simulink model "SerialWriteText"  (R2018a)
settings: Solver=FixedStepAuto  StartTime=0.0  StopTime=5  FixedStep=.1  RelTol=1e-3
libraries: arduinolib x1
settings Model: ExtModeTrigDuration=2  Creator=jonathancoulter  LastModifiedBy=jonathancoulter
settings OptimizationCC: UseFloatMulNetSlope=on  PassReuseOutputArgsThreshold=0  EfficientFloat2IntCast=on  MaxStackSize=64
settings DebuggingCC: ParameterTunabilityLossMsg=error
settings HardwareCC: ProdBitPerInt=16  ProdBitPerPointer=16  ProdBitPerSizeT=16  ProdBitPerPtrDiffT=16  ProdLargestAtomicFloat=None  ProdWordSize=8  ProdHWDeviceType=Atmel->AVR  UseEmbeddedCoderFeatures=off
settings ModelReferenceCC: ModelReferenceMinAlgLoopOccurrences=on
settings SFSimCC: MATLABDynamicMemAlloc=off
settings RTWCC: SystemTargetFile=ert.tlc  HardwareBoard=Arduino Mega 2560  TLCOptions=-aInlineSetEventsForThisBaseRateFcn=TLC_FALSE -aSuppressMultiTaskScheduler=TLC_FALSE -aRateBasedStepFcn=1  TemplateMakefile=ert_default_tmf  Toolchain=Arduino AVR  BuildConfiguration=Faster Runs
settings CodeAppCC: ForceParamTrailComments=on  OperatorAnnotations=on  StateflowObjectComments=on  MATLABSourceComments=on
settings ERTTargetCC: ERTCustomFileBanners=off  SupportContinuousTime=on  SupportNonInlinedSFcns=on  RemoveResetFunc=off  SupportVariableSizeSignals=on  ModelStepFunctionPrototypeControlCompliant=off

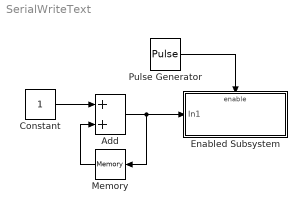
== system SerialWriteText ==
  Add : Sum
  Constant : Constant
  Enabled Subsystem : Subsystem  TreatAsAtomicUnit=on
  Memory : Memory
  Pulse Generator : DiscretePulseGenerator  PulseType=Time based  Period=1  PulseWidth=50
  wires:
  Pulse Generator/1 -> Enabled Subsystem/Enable
  Constant/1 -> Add/1
  Add/1 -> Memory/1, Enabled Subsystem/1(In1)
  Memory/1 -> Add/2

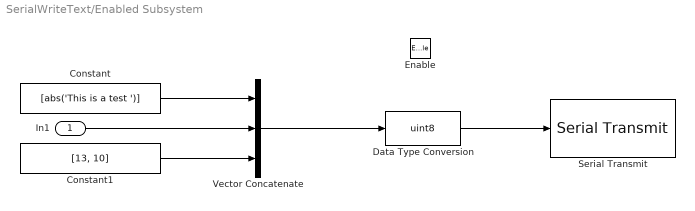
== system SerialWriteText/Enabled Subsystem ==
  In1 : Inport
  Enable : EnablePort
  Constant : Constant  Value=[abs('This is a test ')]
  Constant1 : Constant  Value=[13, 10]
  Data Type Conversion : DataTypeConversion  OutDataTypeStr=uint8
  Serial Transmit : arduinolib/Serial Transmit  portNumber=0  sendmode=write  label=Steering Wheel Position:  sendformat=Decimal  floatprecision=2  blockPlatform=arduino
      settings: SourceProductName=Simulink Support Package for Arduino Hardware
  Vector Concatenate : Concatenate  NumInputs=3
  wires:
  Vector Concatenate/1 -> Data Type Conversion/1
  Data Type Conversion/1 -> Serial Transmit/1
  Constant/1 -> Vector Concatenate/1
  Constant1/1 -> Vector Concatenate/3
  In1/1 -> Vector Concatenate/2
